simulink subsystem "Power_Consumption_clc"  (R2021b)
settings: Solver=VariableStepAuto  StartTime=0.0  StopTime=10.0  RelTol=1e-3
values from neighbouring files (symbols this model uses):
  eff = [0.6437 0.7133 0.7364 0.747 0.7543 0.7657 0.77 0.7708 0.7756 0.7814 0.5842 0.7048 ... (110 elements, 10x11)]    [efficientmap2.mat]
  rev = [500 1000 2000 3000 4000 6000 10000 12000 15000 19000]    [efficientmap2.mat]
  trq = [1.3 2.7 5.4 7.9 10.4 12.5 14.4 16 17.4 18.5 19.6]    [efficientmap2.mat]
settings Model: Creator=tsuyoshi  LastModifiedBy=tsuyoshi

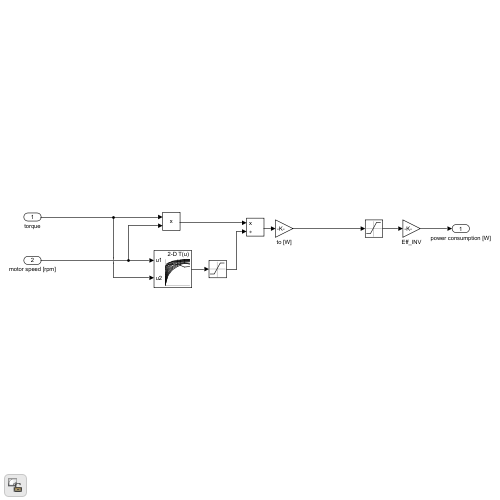
[thumbnail: Simulink's stored preview of the top-level diagram]
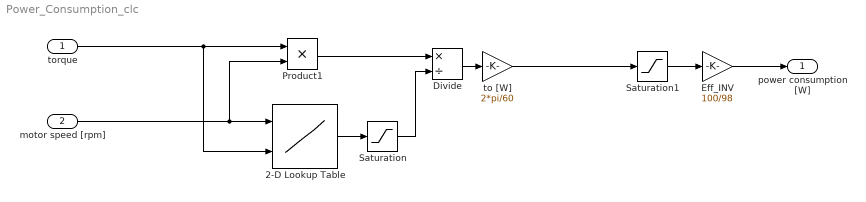
== system Power_Consumption_clc ==
  torque : Inport
  motor speed [rpm] : Inport  Port=2
  2-D Lookup Table : Lookup_n-D  BreakpointsForDimension1=rev  BreakpointsForDimension2=trq  Table=eff  InternalRulePriority=Speed  RndMeth=Simplest  InputSameDT=on
      settings: InputPortMap=u0,u1
  Divide : Product  Inputs=*/
  Eff_INV : Gain  Gain=100/98
  Product1 : Product
  Saturation : Saturate  UpperLimit=1  LowerLimit=0.01
  Saturation1 : Saturate  UpperLimit=35e3  LowerLimit=-35e3
  to [W] : Gain  Gain=2*pi/60
  power consumption [W] : Outport  VectorParamsAs1DForOutWhenUnconnected=off
  wires:
  Product1/1 -> Divide/1
  2-D Lookup Table/1 -> Saturation/1
  Saturation/1 -> Divide/2
  motor speed [rpm]/1 -> 2-D Lookup Table/1, Product1/2
  torque/1 -> 2-D Lookup Table/2, Product1/1
  to [W]/1 -> Saturation1/1
  Eff_INV/1 -> power consumption [W]/1
  Divide/1 -> to [W]/1
  Saturation1/1 -> Eff_INV/1
